simulink model "mrefrobotarm_previous_y_previous_u_previous_ref_cex_3b"  (R2018b)
settings: Solver=FixedStepAuto  StartTime=0.0  StopTime=20  RelTol=1e-3  AbsTol=1e-6
undefined symbols (not defined in the file or in its folder): cc, options
libraries: neural x462, simulink x2
(part 14 of 18)

== system mrefrobotarm_previous_y_previous_u_previous_ref_cex_3b/cex_m5/Layer 3/Delays 1 ==
  "p{3}" : Inport  PortDimensions=30
      mask Display: e = 0.06;c1 = [120 230 180]/255;c2 = ([120 230 180]+0)/(256+128);c3 = ([120 230 180]+128)/(256+128);patch([0 1 1 0],[0 0 1 1],c1);patch([0 1 1 1-e 1-e 0+e],[0 0 1 1-e 0+e 0+e],c2);patch([0 0 1 1-e 0+e 0+e],[0 1 1 1-e 1-e 0+e],c3);plot([0 1 1 0 0],[0 0 1 1 0]);
  mux : Mux  Inputs=1
      mask Display: e = 0.06;c1 = [120 150 230]/255;c2 = ([120 150 230]+0)/383;c3 = ([120 150 230]+128)/383;patch([0 1 1 0],[0 0 1 1],c1);patch([0 1 1 1-e 1-e 0+e],[0 0 1 1-e 0+e 0+e],c2);patch([0 0 1 1-e 0+e 0+e],[0 1 1 1-e 1-e 0+e],c3);plot([0 1 1 0 0],[0 0 1 1 0]);disp('Mux')
  "pd{3,2}" : Outport
      mask Display: e = 0.06;c1 = [120 230 180]/255;c2 = ([120 230 180]+0)/(256+128);c3 = ([120 230 180]+128)/(256+128);patch([0 1 1 0],[0 0 1 1],c1);patch([0 1 1 1-e 1-e 0+e],[0 0 1 1-e 0+e 0+e],c2);patch([0 0 1 1-e 0+e 0+e],[0 1 1 1-e 1-e 0+e],c3);plot([0 1 1 0 0],[0 0 1 1 0]);
  wires:
  "p{3}"/1 -> mux/1
  mux/1 -> "pd{3,2}"/1

== system mrefrobotarm_previous_y_previous_u_previous_ref_cex_3b/cex_m5/Layer 3/LW{3,2} ==
  "ad{3,2}" : Inport  PortDimensions=30
      mask Display: e = 0.06;c1 = [120 230 180]/255;c2 = ([120 230 180]+0)/(256+128);c3 = ([120 230 180]+128)/(256+128);patch([0 1 1 0],[0 0 1 1],c1);patch([0 1 1 1-e 1-e 0+e],[0 0 1 1-e 0+e 0+e],c2);patch([0 0 1 1-e 0+e 0+e],[0 1 1 1-e 1-e 0+e],c3);plot([0 1 1 0 0],[0 0 1 1 0]);
  "IW{3,2}(1,:)'" : Constant  Value=[0.50803666019963544808746291892020963132381439208984375;-0.729030644030080221540401907986961305141448974609375;0.09247581248743631798792108611451112665235996246337890625;-0.034331210467475899161815533489061635918915271759033203125;0.486684870445886763601350821772939525544643402099609375;0.7990123045007149205076757425558753311634063720703125;0.1682973469083234030474471865090890787541866302490234375;-0.474890180914950443824551484794938005506992340087890625;0.270457873152577799036322403480880893766880035400390625;-0.130728690312984008325969398356392048299312591552734375;-0.63017565134821751371418940834701061248779296875;0.28365242499360399097696472381358034908771514892578125;-0.11891322983694736781234979616783675737679004669189453125;0.444577906739277384229325207343208603560924530029296875;0.1091866209193628478590909480772097595036029815673828125;0.126623611089255960759913932633935473859310150146484375;0.88512666352133007041658174784970469772815704345703125;0.478777881050120923678292683689505793154239654541015625;0.4064587284632479313728481429279781877994537353515625;-0.317131905106795730642232911122846417129039764404296875;-0.7472199432531414498015465142088942229747772216796875;-0.7716850440813833866826598750776611268520355224609375;0.07278752047878193909280497564395773224532604217529296875;-0.12570824626491206021938751291600055992603302001953125;-0.2066677692862751436475576838347478769719600677490234375;0.8641321421683898496013398471404798328876495361328125;0.29316217307002201408749897382222115993499755859375;0.348121183619366003636486084360512904822826385498046875;0.10311848126639755474087678521755151450634002685546875;0.77075459933333989592796342549263499677181243896484375]
      mask Display: e = 0.06;c1 = [120 150 230]/255;c2 = ([120 150 230]+0)/383;c3 = ([120 150 230]+128)/383;patch([0 1 1 0],[0 0 1 1],c1);patch([0 1 1 1-e 1-e 0+e],[0 0 1 1-e 0+e 0+e],c2);patch([0 0 1 1-e 0+e 0+e],[0 1 1 1-e 1-e 0+e],c3);plot([0 1 1 0 0],[0 0 1 1 0]);disp('weights');
  Mux : Mux  Inputs=1
      mask Display: e = 0.06;c1 = [120 150 230]/255;c2 = ([120 150 230]+0)/383;c3 = ([120 150 230]+128)/383;patch([0 1 1 0],[0 0 1 1],c1);patch([0 1 1 1-e 1-e 0+e],[0 0 1 1-e 0+e 0+e],c2);patch([0 0 1 1-e 0+e 0+e],[0 1 1 1-e 1-e 0+e],c3);plot([0 1 1 0 0],[0 0 1 1 0]);disp('Mux');
  dotprod1 : neural/Weight Functions/dotprod
  "lz{3,2}" : Outport
      mask Display: e = 0.06;c1 = [120 230 180]/255;c2 = ([120 230 180]+0)/(256+128);c3 = ([120 230 180]+128)/(256+128);patch([0 1 1 0],[0 0 1 1],c1);patch([0 1 1 1-e 1-e 0+e],[0 0 1 1-e 0+e 0+e],c2);patch([0 0 1 1-e 0+e 0+e],[0 1 1 1-e 1-e 0+e],c3);plot([0 1 1 0 0],[0 0 1 1 0]);
  wires:
  "IW{3,2}(1,:)'"/1 -> dotprod1/1
  "ad{3,2}"/1 -> dotprod1/2
  dotprod1/1 -> Mux/1
  Mux/1 -> "lz{3,2}"/1

== system mrefrobotarm_previous_y_previous_u_previous_ref_cex_3b/no_cex/Layer 1/Delays 1 ==
  "p{1}" : Inport  PortDimensions=10
      mask Display: e = 0.06;c1 = [120 230 180]/255;c2 = ([120 230 180]+0)/(256+128);c3 = ([120 230 180]+128)/(256+128);patch([0 1 1 0],[0 0 1 1],c1);patch([0 1 1 1-e 1-e 0+e],[0 0 1 1-e 0+e 0+e],c2);patch([0 0 1 1-e 0+e 0+e],[0 1 1 1-e 1-e 0+e],c3);plot([0 1 1 0 0],[0 0 1 1 0]);
  mux : Mux  Inputs=1
      mask Display: e = 0.06;c1 = [120 150 230]/255;c2 = ([120 150 230]+0)/383;c3 = ([120 150 230]+128)/383;patch([0 1 1 0],[0 0 1 1],c1);patch([0 1 1 1-e 1-e 0+e],[0 0 1 1-e 0+e 0+e],c2);patch([0 0 1 1-e 0+e 0+e],[0 1 1 1-e 1-e 0+e],c3);plot([0 1 1 0 0],[0 0 1 1 0]);disp('Mux')
  "pd{1,1}" : Outport
      mask Display: e = 0.06;c1 = [120 230 180]/255;c2 = ([120 230 180]+0)/(256+128);c3 = ([120 230 180]+128)/(256+128);patch([0 1 1 0],[0 0 1 1],c1);patch([0 1 1 1-e 1-e 0+e],[0 0 1 1-e 0+e 0+e],c2);patch([0 0 1 1-e 0+e 0+e],[0 1 1 1-e 1-e 0+e],c3);plot([0 1 1 0 0],[0 0 1 1 0]);
  wires:
  "p{1}"/1 -> mux/1
  mux/1 -> "pd{1,1}"/1

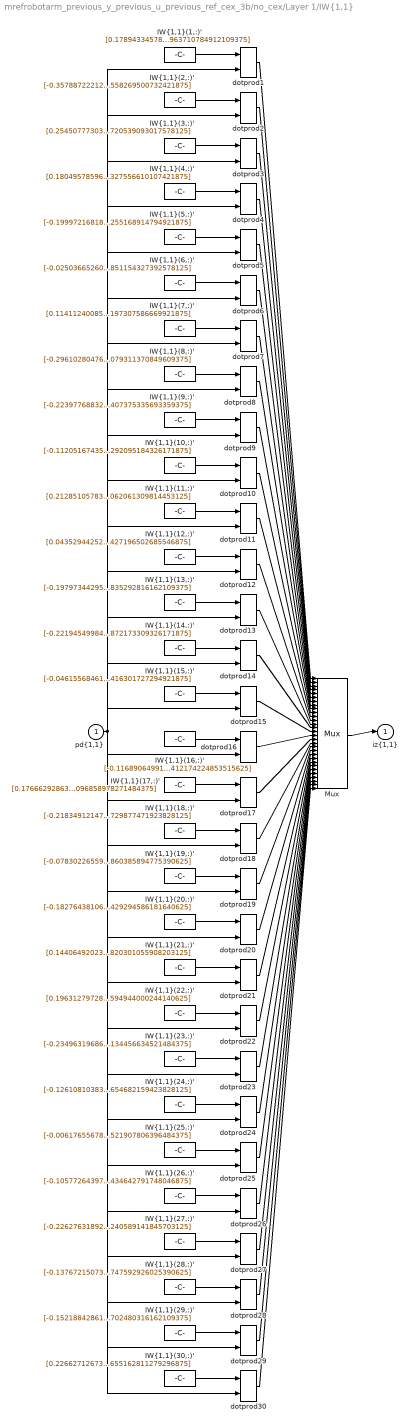
== system mrefrobotarm_previous_y_previous_u_previous_ref_cex_3b/no_cex/Layer 1/IW{1,1} ==
  "pd{1,1}" : Inport  PortDimensions=10
      mask Display: e = 0.06;c1 = [120 230 180]/255;c2 = ([120 230 180]+0)/(256+128);c3 = ([120 230 180]+128)/(256+128);patch([0 1 1 0],[0 0 1 1],c1);patch([0 1 1 1-e 1-e 0+e],[0 0 1 1-e 0+e 0+e],c2);patch([0 0 1 1-e 0+e 0+e],[0 1 1 1-e 1-e 0+e],c3);plot([0 1 1 0 0],[0 0 1 1 0]);
  "IW{1,1}(1,:)'" : Constant  Value=[0.1789433457845766017868527342216111719608306884765625;0.026806665156776932068538599196472205221652984619140625;-0.019425018864830494169648744673395412974059581756591796875;-0.08160374694861978472903984993536141701042652130126953125;-0.09141214122166922695367219375839340500533580780029296875;-0.0300317987322644870673560291152170975692570209503173828125;-0.28242027541455028138983607277623377740383148193359375;0.131111008237114468055750649000401608645915985107421875;-0.1895896042370200651472345043657696805894374847412109375;0.2425039454857501330931057736961520276963710784912109375]
      mask Display: e = 0.06;c1 = [120 150 230]/255;c2 = ([120 150 230]+0)/383;c3 = ([120 150 230]+128)/383;patch([0 1 1 0],[0 0 1 1],c1);patch([0 1 1 1-e 1-e 0+e],[0 0 1 1-e 0+e 0+e],c2);patch([0 0 1 1-e 0+e 0+e],[0 1 1 1-e 1-e 0+e],c3);plot([0 1 1 0 0],[0 0 1 1 0]);disp('Weights');
  "IW{1,1}(10,:)'" : Constant  Value=[-0.11205167435669681486043458562562591396272182464599609375;0.3571497785474593289478661972680129110813140869140625;-0.2471594181194160799730497046766686253249645233154296875;0.0269727210263034818116256730036184308119118213653564453125;0.333375233420288186181323908385820686817169189453125;-0.3923415376813588206772465127869509160518646240234375;0.10451408189524002967374372019548900425434112548828125;-0.06697052425982270851267941225160029716789722442626953125;-0.08640964459355114646310624948455370031297206878662109375;-0.39109382895870126173321068563382141292095184326171875]
      mask Display: e = 0.06;c1 = [120 150 230]/255;c2 = ([120 150 230]+0)/383;c3 = ([120 150 230]+128)/383;patch([0 1 1 0],[0 0 1 1],c1);patch([0 1 1 1-e 1-e 0+e],[0 0 1 1-e 0+e 0+e],c2);patch([0 0 1 1-e 0+e 0+e],[0 1 1 1-e 1-e 0+e],c3);plot([0 1 1 0 0],[0 0 1 1 0]);disp('Weights');
  "IW{1,1}(11,:)'" : Constant  Value=[0.2128510578334973646352779041990288533270359039306640625;-0.202231663792214522157308920213836245238780975341796875;0.0248759940897357034739201253614737652242183685302734375;-0.15238132615766508681787172463373281061649322509765625;0.01341935499692491380596681693759819609113037586212158203125;0.333773414996746620175827047205530107021331787109375;-0.12205302921810114169520744553665281273424625396728515625;0.154445274700418855307049170733080245554447174072265625;-0.0299658607885634718781542318311039707623422145843505859375;0.1513989913513389684585064287603017874062061309814453125]
      mask Display: e = 0.06;c1 = [120 150 230]/255;c2 = ([120 150 230]+0)/383;c3 = ([120 150 230]+128)/383;patch([0 1 1 0],[0 0 1 1],c1);patch([0 1 1 1-e 1-e 0+e],[0 0 1 1-e 0+e 0+e],c2);patch([0 0 1 1-e 0+e 0+e],[0 1 1 1-e 1-e 0+e],c3);plot([0 1 1 0 0],[0 0 1 1 0]);disp('Weights');
  "IW{1,1}(12,:)'" : Constant  Value=[0.04352944252029027072392608488371479324996471405029296875;-0.4145342324684342383278590205009095370769500732421875;0.215269820769206976507348372251726686954498291015625;0.16656367985601061576517167850397527217864990234375;-0.023581251549110941734266333469349774532020092010498046875;0.08572964794493535822805796442480641417205333709716796875;-0.1958135172033455273510327288022381253540515899658203125;-0.1625056502497410904073404935843427665531635284423828125;0.251217425233158042630066120182164013385772705078125;-0.1069272106474794536978834003093652427196502685546875]
      mask Display: e = 0.06;c1 = [120 150 230]/255;c2 = ([120 150 230]+0)/383;c3 = ([120 150 230]+128)/383;patch([0 1 1 0],[0 0 1 1],c1);patch([0 1 1 1-e 1-e 0+e],[0 0 1 1-e 0+e 0+e],c2);patch([0 0 1 1-e 0+e 0+e],[0 1 1 1-e 1-e 0+e],c3);plot([0 1 1 0 0],[0 0 1 1 0]);disp('Weights');
  "IW{1,1}(13,:)'" : Constant  Value=[-0.1979734429534960316043878947311895899474620819091796875;0.184541564617396514069724844375741668045520782470703125;-0.0638366095873931505000342667699442245066165924072265625;0.2121216584407361882558262777820345945656299591064453125;-0.1380891994715965076512276255016331560909748077392578125;0.038970800909377711906955710219335742294788360595703125;0.1056185799492942722910271413638838566839694976806640625;-0.150221719826857891266769229332567192614078521728515625;-0.2463272007812304931206881519756279885768890380859375;0.217176977670956394828039037747657857835292816162109375]
      mask Display: e = 0.06;c1 = [120 150 230]/255;c2 = ([120 150 230]+0)/383;c3 = ([120 150 230]+128)/383;patch([0 1 1 0],[0 0 1 1],c1);patch([0 1 1 1-e 1-e 0+e],[0 0 1 1-e 0+e 0+e],c2);patch([0 0 1 1-e 0+e 0+e],[0 1 1 1-e 1-e 0+e],c3);plot([0 1 1 0 0],[0 0 1 1 0]);disp('Weights');
  "IW{1,1}(14,:)'" : Constant  Value=[-0.2219454998402757561759557347613736055791378021240234375;-0.03146157022389335644607655240179155953228473663330078125;0.251007319128800698848635875037871301174163818359375;-0.0716759659946031302268920626374892890453338623046875;-0.0172769424599281511134574174093359033577144145965576171875;0.187315939375391149468441653880290687084197998046875;0.1900738665719299003153963667500647716224193572998046875;0.256287588268780563982573994508129544556140899658203125;-0.12311552872518909118593199991664732806384563446044921875;0.083687737575868836881198831179062835872173309326171875]
      mask Display: e = 0.06;c1 = [120 150 230]/255;c2 = ([120 150 230]+0)/383;c3 = ([120 150 230]+128)/383;patch([0 1 1 0],[0 0 1 1],c1);patch([0 1 1 1-e 1-e 0+e],[0 0 1 1-e 0+e 0+e],c2);patch([0 0 1 1-e 0+e 0+e],[0 1 1 1-e 1-e 0+e],c3);plot([0 1 1 0 0],[0 0 1 1 0]);disp('Weights');
  "IW{1,1}(15,:)'" : Constant  Value=[-0.046155684619317384476122612113613286055624485015869140625;-0.1501347766892376645042617155922926031053066253662109375;0.00923054671975952721607594497754689655266702175140380859375;-0.263036162746853541261060627221013419330120086669921875;-0.232797656826339238733680758741684257984161376953125;-0.20261136681460356623318830315838567912578582763671875;0.051737147633385383027615489481831900775432586669921875;-0.2097569798040830324481476054643280804157257080078125;0.1810701944794087248080671770367189310491085052490234375;-0.037977663494814066502680560688531841151416301727294921875]
      mask Display: e = 0.06;c1 = [120 150 230]/255;c2 = ([120 150 230]+0)/383;c3 = ([120 150 230]+128)/383;patch([0 1 1 0],[0 0 1 1],c1);patch([0 1 1 1-e 1-e 0+e],[0 0 1 1-e 0+e 0+e],c2);patch([0 0 1 1-e 0+e 0+e],[0 1 1 1-e 1-e 0+e],c3);plot([0 1 1 0 0],[0 0 1 1 0]);disp('Weights');
  "IW{1,1}(16,:)'" : Constant  Value=[-0.11689064991597501730336006176003138534724712371826171875;0.1948274101793631418733099280871101655066013336181640625;0.245143937349593776797718192028696648776531219482421875;0.06314433664036896154403422087852959521114826202392578125;-0.1710716489566988240955680566912633366882801055908203125;0.228635751900371164690994874035823158919811248779296875;0.167954804626501530417925778237986378371715545654296875;-0.1360225837338669696574555700863129459321498870849609375;0.1710850798697334529396840707704541273415088653564453125;-0.03517706195236515454016767989742220379412174224853515625]
      mask Display: e = 0.06;c1 = [120 150 230]/255;c2 = ([120 150 230]+0)/383;c3 = ([120 150 230]+128)/383;patch([0 1 1 0],[0 0 1 1],c1);patch([0 1 1 1-e 1-e 0+e],[0 0 1 1-e 0+e 0+e],c2);patch([0 0 1 1-e 0+e 0+e],[0 1 1 1-e 1-e 0+e],c3);plot([0 1 1 0 0],[0 0 1 1 0]);disp('Weights');
  "IW{1,1}(17,:)'" : Constant  Value=[0.1766629286340325732940215175403864122927188873291015625;-0.07924000184714556638265747778859804384410381317138671875;-0.079307885697641300470905889596906490623950958251953125;-0.1959224066965960242558963955161743797361850738525390625;0.1156529952522807602743881716378382407128810882568359375;0.00787969713280355955886680163757773698307573795318603515625;0.042693454259183853671810737751002307049930095672607421875;-0.2093969688941783591218381843646056950092315673828125;-0.1737244673605020661710796048282645642757415771484375;-0.30776382007785529903998167355894111096858978271484375]
      mask Display: e = 0.06;c1 = [120 150 230]/255;c2 = ([120 150 230]+0)/383;c3 = ([120 150 230]+128)/383;patch([0 1 1 0],[0 0 1 1],c1);patch([0 1 1 1-e 1-e 0+e],[0 0 1 1-e 0+e 0+e],c2);patch([0 0 1 1-e 0+e 0+e],[0 1 1 1-e 1-e 0+e],c3);plot([0 1 1 0 0],[0 0 1 1 0]);disp('Weights');
  "IW{1,1}(18,:)'" : Constant  Value=[-0.2183491214766035692917967026005499064922332763671875;0.064228498311528825492899841265170834958553314208984375;-0.061951741605276833269044800545088946819305419921875;0.0980483298401862712889709428054629825055599212646484375;-0.1940715279329147946452138739914516918361186981201171875;0.100554472875109379703673084804904647171497344970703125;0.05512572940682851363458638616066309623420238494873046875;-0.2225697983573027005643751863317447714507579803466796875;0.307695093952117415536662292652181349694728851318359375;0.035102615659615206411547916331983287818729877471923828125]
      mask Display: e = 0.06;c1 = [120 150 230]/255;c2 = ([120 150 230]+0)/383;c3 = ([120 150 230]+128)/383;patch([0 1 1 0],[0 0 1 1],c1);patch([0 1 1 1-e 1-e 0+e],[0 0 1 1-e 0+e 0+e],c2);patch([0 0 1 1-e 0+e 0+e],[0 1 1 1-e 1-e 0+e],c3);plot([0 1 1 0 0],[0 0 1 1 0]);disp('Weights');
  "IW{1,1}(19,:)'" : Constant  Value=[-0.078302265597536335750561420354642905294895172119140625;-0.11015731653471379225539550361645524390041828155517578125;0.070372247422889111501120851244195364415645599365234375;-0.07371385722816987950967160259096999652683734893798828125;0.2498389657291748833234379389978130348026752471923828125;-0.14478671437019630108267165269353426992893218994140625;0.3213022509194900511175774227012880146503448486328125;0.014213136324984949887539897872557048685848712921142578125;-0.209759210724774380896207048863288946449756622314453125;-0.13789802555820040996792386067681945860385894775390625]
      mask Display: e = 0.06;c1 = [120 150 230]/255;c2 = ([120 150 230]+0)/383;c3 = ([120 150 230]+128)/383;patch([0 1 1 0],[0 0 1 1],c1);patch([0 1 1 1-e 1-e 0+e],[0 0 1 1-e 0+e 0+e],c2);patch([0 0 1 1-e 0+e 0+e],[0 1 1 1-e 1-e 0+e],c3);plot([0 1 1 0 0],[0 0 1 1 0]);disp('Weights');
  "IW{1,1}(2,:)'" : Constant  Value=[-0.357887222121373971273072811527526937425136566162109375;-0.1701508970623704930513753197374171577394008636474609375;0.1283995799451636832255729814278311096131801605224609375;0.027882319431207010229645248955421266146004199981689453125;0.2413367899208160860524685631389729678630828857421875;-0.08829939749269695437039473517870646901428699493408203125;-0.059645223459835527979322478131507523357868194580078125;-0.1817708312802679693209739753001485951244831085205078125;-0.202751405688736785482007007885840721428394317626953125;0.036121615813504197312067134362223441712558269500732421875]
      mask Display: e = 0.06;c1 = [120 150 230]/255;c2 = ([120 150 230]+0)/383;c3 = ([120 150 230]+128)/383;patch([0 1 1 0],[0 0 1 1],c1);patch([0 1 1 1-e 1-e 0+e],[0 0 1 1-e 0+e 0+e],c2);patch([0 0 1 1-e 0+e 0+e],[0 1 1 1-e 1-e 0+e],c3);plot([0 1 1 0 0],[0 0 1 1 0]);disp('Weights');
  "IW{1,1}(20,:)'" : Constant  Value=[-0.1827643810609429209090848189589451067149639129638671875;0.429780420918997874135669690076611004769802093505859375;0.04752296112356881041538514409694471396505832672119140625;-0.051704435533531163671217001365221221931278705596923828125;0.09194866005832495747807087127512204460799694061279296875;-0.378826441233361788096800637504202313721179962158203125;-0.032643642152327199956740599873228347860276699066162109375;-0.035924345859773477995791068906328291632235050201416015625;-0.0821961773385673499792147822518018074333667755126953125;-0.1229117568782160108131762399352737702429294586181640625]
      mask Display: e = 0.06;c1 = [120 150 230]/255;c2 = ([120 150 230]+0)/383;c3 = ([120 150 230]+128)/383;patch([0 1 1 0],[0 0 1 1],c1);patch([0 1 1 1-e 1-e 0+e],[0 0 1 1-e 0+e 0+e],c2);patch([0 0 1 1-e 0+e 0+e],[0 1 1 1-e 1-e 0+e],c3);plot([0 1 1 0 0],[0 0 1 1 0]);disp('Weights');
  "IW{1,1}(21,:)'" : Constant  Value=[0.144064920235662696779144198444555513560771942138671875;0.056739780550756180321769761576433666050434112548828125;0.1869901994016132940057417499701841734349727630615234375;-0.1647949003581190841050130302392062731087207794189453125;-0.237382679487966596898473881083191372454166412353515625;0.25368592107000653701476267087855376303195953369140625;-0.234657572045289197770756572936079464852809906005859375;0.021587502157350169085248126066289842128753662109375;0.23838937978631380421035146355279721319675445556640625;-0.002599061752152885713951224744278079015202820301055908203125]
      mask Display: e = 0.06;c1 = [120 150 230]/255;c2 = ([120 150 230]+0)/383;c3 = ([120 150 230]+128)/383;patch([0 1 1 0],[0 0 1 1],c1);patch([0 1 1 1-e 1-e 0+e],[0 0 1 1-e 0+e 0+e],c2);patch([0 0 1 1-e 0+e 0+e],[0 1 1 1-e 1-e 0+e],c3);plot([0 1 1 0 0],[0 0 1 1 0]);disp('Weights');
  "IW{1,1}(22,:)'" : Constant  Value=[0.196312797288851148547195180071867071092128753662109375;-0.052003440136825181128177320033501018770039081573486328125;-0.271537484269043394302656224681413732469081878662109375;-0.08952689103963186456613954078420647419989109039306640625;-0.03695367511956813844076208397382288239896297454833984375;0.00447587075779976202583032574011667747981846332550048828125;0.2592011849893742780892580412910319864749908447265625;-0.088946395220038609874535495691816322505474090576171875;0.0322691823643851682934524660595343448221683502197265625;0.30695137976644348842825138490297831594944000244140625]
      mask Display: e = 0.06;c1 = [120 150 230]/255;c2 = ([120 150 230]+0)/383;c3 = ([120 150 230]+128)/383;patch([0 1 1 0],[0 0 1 1],c1);patch([0 1 1 1-e 1-e 0+e],[0 0 1 1-e 0+e 0+e],c2);patch([0 0 1 1-e 0+e 0+e],[0 1 1 1-e 1-e 0+e],c3);plot([0 1 1 0 0],[0 0 1 1 0]);disp('Weights');
  "IW{1,1}(23,:)'" : Constant  Value=[-0.2349631968647795388083210355034680105745792388916015625;-0.1764143763037677448135553959218668751418590545654296875;0.2349121078796777284392049978123395703732967376708984375;0.09797592905204242919037227466105832718312740325927734375;0.27541249925572675039120440487749874591827392578125;-0.00667307854933686661613734258935437537729740142822265625;-0.0863088887077549105075746638249256648123264312744140625;-0.049254487681551224753651041510238428600132465362548828125;0.3119811716961577996443111260305158793926239013671875;-0.1301709247348719900028157780980109237134456634521484375]
      mask Display: e = 0.06;c1 = [120 150 230]/255;c2 = ([120 150 230]+0)/383;c3 = ([120 150 230]+128)/383;patch([0 1 1 0],[0 0 1 1],c1);patch([0 1 1 1-e 1-e 0+e],[0 0 1 1-e 0+e 0+e],c2);patch([0 0 1 1-e 0+e 0+e],[0 1 1 1-e 1-e 0+e],c3);plot([0 1 1 0 0],[0 0 1 1 0]);disp('Weights');
  "IW{1,1}(24,:)'" : Constant  Value=[-0.126108103838845353461550757856457494199275970458984375;0.08453501177616129513836540354532189667224884033203125;-0.1709620737039248272726155164491501636803150177001953125;0.291184483266852811578218052090960554778575897216796875;0.11522387540724605969888472145612468011677265167236328125;0.27025016099325138707598625842365436255931854248046875;0.115017676269625723772804803957114927470684051513671875;0.06893159212255894896514973879675380885601043701171875;0.09231217475138053796257509020506404340267181396484375;0.1257462335265127351124903043455560691654682159423828125]
      mask Display: e = 0.06;c1 = [120 150 230]/255;c2 = ([120 150 230]+0)/383;c3 = ([120 150 230]+128)/383;patch([0 1 1 0],[0 0 1 1],c1);patch([0 1 1 1-e 1-e 0+e],[0 0 1 1-e 0+e 0+e],c2);patch([0 0 1 1-e 0+e 0+e],[0 1 1 1-e 1-e 0+e],c3);plot([0 1 1 0 0],[0 0 1 1 0]);disp('Weights');
  "IW{1,1}(25,:)'" : Constant  Value=[-0.00617655678054580652147631525394899654202163219451904296875;0.158550050715132895273740132324746809899806976318359375;0.18860048113506466815891826627193950116634368896484375;-0.016879223596091640080540940971332020126283168792724609375;-0.1887910208933633315897537841010489501059055328369140625;0.1272457432851887559888126588703016750514507293701171875;-0.018568139538292789680884453673570533283054828643798828125;0.2719728918008812446061028822441585361957550048828125;0.1140621157238612404238864428407396189868450164794921875;-0.2380940842603967710910950472680269740521907806396484375]
      mask Display: e = 0.06;c1 = [120 150 230]/255;c2 = ([120 150 230]+0)/383;c3 = ([120 150 230]+128)/383;patch([0 1 1 0],[0 0 1 1],c1);patch([0 1 1 1-e 1-e 0+e],[0 0 1 1-e 0+e 0+e],c2);patch([0 0 1 1-e 0+e 0+e],[0 1 1 1-e 1-e 0+e],c3);plot([0 1 1 0 0],[0 0 1 1 0]);disp('Weights');
  "IW{1,1}(26,:)'" : Constant  Value=[-0.105772643970521940115503412016551010310649871826171875;0.1782055718246454978359594178982661105692386627197265625;-0.257768734053310577536421988043002784252166748046875;-0.12118741242321341700094450288816005922853946685791015625;0.10799318799709652083596012062116642482578754425048828125;0.032415029855224826438320206989374128170311450958251953125;0.23392792477851431787172487020143307745456695556640625;0.048627216784484859901649400626411079429090023040771484375;-0.07777159955391781120948024863537284545600414276123046875;-0.066068946728559563297267231973819434642791748046875]
      mask Display: e = 0.06;c1 = [120 150 230]/255;c2 = ([120 150 230]+0)/383;c3 = ([120 150 230]+128)/383;patch([0 1 1 0],[0 0 1 1],c1);patch([0 1 1 1-e 1-e 0+e],[0 0 1 1-e 0+e 0+e],c2);patch([0 0 1 1-e 0+e 0+e],[0 1 1 1-e 1-e 0+e],c3);plot([0 1 1 0 0],[0 0 1 1 0]);disp('Weights');
  "IW{1,1}(27,:)'" : Constant  Value=[-0.2262763189227159077443474188839900307357311248779296875;0.2283819320597203772482686190414824523031711578369140625;-0.046330569948930359902572462260650354437530040740966796875;-0.21556632228014915853009370039217174053192138671875;-0.024471900852634960454867751877827686257660388946533203125;-0.061310669133914065531687498378232703544199466705322265625;0.1926380354105947934062470494609442539513111114501953125;0.2138008717117891588355149679046007804572582244873046875;0.2402187286512235953050975467704120092093944549560546875;0.004683890847436260503056093540408255648799240589141845703125]
      mask Display: e = 0.06;c1 = [120 150 230]/255;c2 = ([120 150 230]+0)/383;c3 = ([120 150 230]+128)/383;patch([0 1 1 0],[0 0 1 1],c1);patch([0 1 1 1-e 1-e 0+e],[0 0 1 1-e 0+e 0+e],c2);patch([0 0 1 1-e 0+e 0+e],[0 1 1 1-e 1-e 0+e],c3);plot([0 1 1 0 0],[0 0 1 1 0]);disp('Weights');
  "IW{1,1}(28,:)'" : Constant  Value=[-0.1376721507398574739777785680416855029761791229248046875;0.1357305892334177144231688316722284071147441864013671875;0.10902662094067107345640721405288786627352237701416015625;-0.0209302692967432597825894191601037164218723773956298828125;0.1596193252357711311884003180239233188331127166748046875;-0.22463253929018323074018326224177144467830657958984375;-0.126742784051142420853608427933068014681339263916015625;0.1520246488067715506797838997954386286437511444091796875;0.2181396982129823192142481502742157317698001861572265625;-0.0472266865883811670645542335478239692747592926025390625]
      mask Display: e = 0.06;c1 = [120 150 230]/255;c2 = ([120 150 230]+0)/383;c3 = ([120 150 230]+128)/383;patch([0 1 1 0],[0 0 1 1],c1);patch([0 1 1 1-e 1-e 0+e],[0 0 1 1-e 0+e 0+e],c2);patch([0 0 1 1-e 0+e 0+e],[0 1 1 1-e 1-e 0+e],c3);plot([0 1 1 0 0],[0 0 1 1 0]);disp('Weights');
  "IW{1,1}(29,:)'" : Constant  Value=[-0.1521884286183979029249968561998684890568256378173828125;-0.045825061815970465073366568731216830201447010040283203125;0.075552021378081202218623957378440536558628082275390625;-0.185262385097363424524274932991829700767993927001953125;0.151250917067363932488888167426921427249908447265625;-0.1412092387151698547054223809027462266385555267333984375;-0.08681829974009762362907594024363788776099681854248046875;-0.2248735479200896503204631926564616151154041290283203125;-0.1651995887555126885093415012306650169193744659423828125;0.157553780756952865882425385279930196702480316162109375]
      mask Display: e = 0.06;c1 = [120 150 230]/255;c2 = ([120 150 230]+0)/383;c3 = ([120 150 230]+128)/383;patch([0 1 1 0],[0 0 1 1],c1);patch([0 1 1 1-e 1-e 0+e],[0 0 1 1-e 0+e 0+e],c2);patch([0 0 1 1-e 0+e 0+e],[0 1 1 1-e 1-e 0+e],c3);plot([0 1 1 0 0],[0 0 1 1 0]);disp('Weights');
  "IW{1,1}(3,:)'" : Constant  Value=[0.2545077730308322738750348435132764279842376708984375;0.040200772337387093158245221502511412836611270904541015625;0.1688552759835511007935338056995533406734466552734375;0.2275439474123589767007302953061298467218875885009765625;0.238416378071425294482565959697240032255649566650390625;0.1413290648624935530452972898274310864508152008056640625;0.1057585717371296307742767339732381515204906463623046875;0.1334076779718362526505615051064523868262767791748046875;0.120305182199565041667455034257727675139904022216796875;0.11598616375682953283376974695784156210720539093017578125]
      mask Display: e = 0.06;c1 = [120 150 230]/255;c2 = ([120 150 230]+0)/383;c3 = ([120 150 230]+128)/383;patch([0 1 1 0],[0 0 1 1],c1);patch([0 1 1 1-e 1-e 0+e],[0 0 1 1-e 0+e 0+e],c2);patch([0 0 1 1-e 0+e 0+e],[0 1 1 1-e 1-e 0+e],c3);plot([0 1 1 0 0],[0 0 1 1 0]);disp('Weights');
  "IW{1,1}(30,:)'" : Constant  Value=[0.2266271267387724719366559611444245092570781707763671875;0.1400905747425138792028320722238277085125446319580078125;-0.1118692708200293151055149110106867738068103790283203125;0.20125294810015048607709786665509454905986785888671875;-0.0186267634903538349677720731278895982541143894195556640625;-0.200639624098857660694505966603173874318599700927734375;-0.09615771229638904460390591566465445794165134429931640625;-0.177214543927699696990174516031402163207530975341796875;0.03191830542659655767234738732440746389329433441162109375;0.2669655305019122959464539235341362655162811279296875]
      mask Display: e = 0.06;c1 = [120 150 230]/255;c2 = ([120 150 230]+0)/383;c3 = ([120 150 230]+128)/383;patch([0 1 1 0],[0 0 1 1],c1);patch([0 1 1 1-e 1-e 0+e],[0 0 1 1-e 0+e 0+e],c2);patch([0 0 1 1-e 0+e 0+e],[0 1 1 1-e 1-e 0+e],c3);plot([0 1 1 0 0],[0 0 1 1 0]);disp('Weights');
  "IW{1,1}(4,:)'" : Constant  Value=[0.1804957859696745270383644310641102492809295654296875;-0.2288584972184532217998054193230927921831607818603515625;0.1818629338165111963832032415666617453098297119140625;-0.037952073411335406072364406782071455381810665130615234375;-0.00539871852212082947719551384579972364008426666259765625;0.182786368740827043222196834904025308787822723388671875;-0.055300908131749697271839494305822881869971752166748046875;-0.1474442788239329893418272376948152668774127960205078125;-0.27933026497486468375797130647697485983371734619140625;0.132250800721111338997815209950204007327556610107421875]
      mask Display: e = 0.06;c1 = [120 150 230]/255;c2 = ([120 150 230]+0)/383;c3 = ([120 150 230]+128)/383;patch([0 1 1 0],[0 0 1 1],c1);patch([0 1 1 1-e 1-e 0+e],[0 0 1 1-e 0+e 0+e],c2);patch([0 0 1 1-e 0+e 0+e],[0 1 1 1-e 1-e 0+e],c3);plot([0 1 1 0 0],[0 0 1 1 0]);disp('Weights');
  "IW{1,1}(5,:)'" : Constant  Value=[-0.19997216818005469907149063146789558231830596923828125;-0.1629615728772902116805454397763242013752460479736328125;-0.1088061302365657123658593263826332986354827880859375;0.051130930700108122299862856152685708366334438323974609375;-0.023722808228792462148515340913945692591369152069091796875;0.05171942315686968438814830051342141814529895782470703125;-0.172023141245443100810774694764404557645320892333984375;-0.2044816274455876214943828017567284405231475830078125;0.166303750238228686963992686287383548915386199951171875;-0.139186544766161268693593910938943736255168914794921875]
      mask Display: e = 0.06;c1 = [120 150 230]/255;c2 = ([120 150 230]+0)/383;c3 = ([120 150 230]+128)/383;patch([0 1 1 0],[0 0 1 1],c1);patch([0 1 1 1-e 1-e 0+e],[0 0 1 1-e 0+e 0+e],c2);patch([0 0 1 1-e 0+e 0+e],[0 1 1 1-e 1-e 0+e],c3);plot([0 1 1 0 0],[0 0 1 1 0]);disp('Weights');
  "IW{1,1}(6,:)'" : Constant  Value=[-0.025036652606763708239778765118899173103272914886474609375;-0.004459660997023274543737958452993552782572805881500244140625;0.06640274816857501261058160935135674662888050079345703125;-0.213061242876234679943792116318945772945880889892578125;0.1292954929203400105119925456165219657123088836669921875;-0.1347784484203936317125993582521914504468441009521484375;-0.2359879168296239171365158426851849071681499481201171875;-0.06529033806976369813668270580819807946681976318359375;-0.1443014597905320772763815284633892588317394256591796875;0.08876780395364276821101867653851513750851154327392578125]
      mask Display: e = 0.06;c1 = [120 150 230]/255;c2 = ([120 150 230]+0)/383;c3 = ([120 150 230]+128)/383;patch([0 1 1 0],[0 0 1 1],c1);patch([0 1 1 1-e 1-e 0+e],[0 0 1 1-e 0+e 0+e],c2);patch([0 0 1 1-e 0+e 0+e],[0 1 1 1-e 1-e 0+e],c3);plot([0 1 1 0 0],[0 0 1 1 0]);disp('Weights');
  "IW{1,1}(7,:)'" : Constant  Value=[0.114112400854734563626635690525290556252002716064453125;-0.0719764852942859356677018922709976322948932647705078125;0.21942076440832936068403569151996634900569915771484375;0.20872027523270497706420201211585663259029388427734375;0.042791134284794786479810824175729067064821720123291015625;0.01219358252673974352120467301574535667896270751953125;0.103149329692884206277625480652204714715480804443359375;0.2155964323288774020515035090284072794020175933837890625;-0.11201445164094690765121953290872625075280666351318359375;0.267689621647867692644240378285758197307586669921875]
      mask Display: e = 0.06;c1 = [120 150 230]/255;c2 = ([120 150 230]+0)/383;c3 = ([120 150 230]+128)/383;patch([0 1 1 0],[0 0 1 1],c1);patch([0 1 1 1-e 1-e 0+e],[0 0 1 1-e 0+e 0+e],c2);patch([0 0 1 1-e 0+e 0+e],[0 1 1 1-e 1-e 0+e],c3);plot([0 1 1 0 0],[0 0 1 1 0]);disp('Weights');
  "IW{1,1}(8,:)'" : Constant  Value=[-0.296102804766170513151024579201475717127323150634765625;-0.074634028193786450255942099829553626477718353271484375;-0.2385550334875161937464582706525106914341449737548828125;-0.205611704822805829717680126123013906180858612060546875;0.0525654127691315142811845362302847206592559814453125;-0.14543344256929569002778634967398829758167266845703125;0.1567883935266303208067029117955826222896575927734375;0.17216661658090737230253353118314407765865325927734375;-0.0903177999287110566672964750978280790150165557861328125;-0.05251414846928435797845935439909226261079311370849609375]
      mask Display: e = 0.06;c1 = [120 150 230]/255;c2 = ([120 150 230]+0)/383;c3 = ([120 150 230]+128)/383;patch([0 1 1 0],[0 0 1 1],c1);patch([0 1 1 1-e 1-e 0+e],[0 0 1 1-e 0+e 0+e],c2);patch([0 0 1 1-e 0+e 0+e],[0 1 1 1-e 1-e 0+e],c3);plot([0 1 1 0 0],[0 0 1 1 0]);disp('Weights');
  "IW{1,1}(9,:)'" : Constant  Value=[-0.223977688326731871892860681327874772250652313232421875;-0.1882936136938099525028889047462143935263156890869140625;-0.0257945746484941167142590501271115499548614025115966796875;0.07815143539481080037223392764644813723862171173095703125;0.03562614155169104013243241979580488987267017364501953125;-0.037321098578910867626934333429744583554565906524658203125;-0.280712738764397007340534173636115156114101409912109375;0.32608983885085562892669486245722509920597076416015625;0.05207556045307785985709614351435448043048381805419921875;-0.017162587892261237099145176898673526011407375335693359375]
      mask Display: e = 0.06;c1 = [120 150 230]/255;c2 = ([120 150 230]+0)/383;c3 = ([120 150 230]+128)/383;patch([0 1 1 0],[0 0 1 1],c1);patch([0 1 1 1-e 1-e 0+e],[0 0 1 1-e 0+e 0+e],c2);patch([0 0 1 1-e 0+e 0+e],[0 1 1 1-e 1-e 0+e],c3);plot([0 1 1 0 0],[0 0 1 1 0]);disp('Weights');
  Mux : Mux  Inputs=30
      mask Display: e = 0.06;c1 = [120 150 230]/255;c2 = ([120 150 230]+0)/383;c3 = ([120 150 230]+128)/383;patch([0 1 1 0],[0 0 1 1],c1);patch([0 1 1 1-e 1-e 0+e],[0 0 1 1-e 0+e 0+e],c2);patch([0 0 1 1-e 0+e 0+e],[0 1 1 1-e 1-e 0+e],c3);plot([0 1 1 0 0],[0 0 1 1 0]);disp('Mux');
  dotprod{1..30} (30 alike) : neural/Weight Functions/dotprod
  "iz{1,1}" : Outport
      mask Display: e = 0.06;c1 = [120 230 180]/255;c2 = ([120 230 180]+0)/(256+128);c3 = ([120 230 180]+128)/(256+128);patch([0 1 1 0],[0 0 1 1],c1);patch([0 1 1 1-e 1-e 0+e],[0 0 1 1-e 0+e 0+e],c2);patch([0 0 1 1-e 0+e 0+e],[0 1 1 1-e 1-e 0+e],c3);plot([0 1 1 0 0],[0 0 1 1 0]);
  wires:
  "IW{1,1}(1,:)'"/1 -> dotprod1/1
  "pd{1,1}"/1 -> dotprod1/2, dotprod2/2, dotprod3/2, dotprod4/2, dotprod5/2, dotprod6/2, dotprod7/2, dotprod8/2, dotprod9/2, dotprod10/2, dotprod11/2, dotprod12/2, dotprod13/2, dotprod14/2, dotprod15/2, dotprod16/2, dotprod17/2, dotprod18/2, dotprod19/2, dotprod20/2, dotprod21/2, dotprod22/2, dotprod23/2, dotprod24/2, dotprod25/2, dotprod26/2, dotprod27/2, dotprod28/2, dotprod29/2, dotprod30/2
  dotprod1/1 -> Mux/1
  "IW{1,1}(2,:)'"/1 -> dotprod2/1
  dotprod2/1 -> Mux/2
  "IW{1,1}(3,:)'"/1 -> dotprod3/1
  dotprod3/1 -> Mux/3
  "IW{1,1}(4,:)'"/1 -> dotprod4/1
  dotprod4/1 -> Mux/4
  "IW{1,1}(5,:)'"/1 -> dotprod5/1
  dotprod5/1 -> Mux/5
  "IW{1,1}(6,:)'"/1 -> dotprod6/1
  dotprod6/1 -> Mux/6
  "IW{1,1}(7,:)'"/1 -> dotprod7/1
  dotprod7/1 -> Mux/7
  "IW{1,1}(8,:)'"/1 -> dotprod8/1
  dotprod8/1 -> Mux/8
  "IW{1,1}(9,:)'"/1 -> dotprod9/1
  dotprod9/1 -> Mux/9
  "IW{1,1}(10,:)'"/1 -> dotprod10/1
  dotprod10/1 -> Mux/10
  "IW{1,1}(11,:)'"/1 -> dotprod11/1
  dotprod11/1 -> Mux/11
  "IW{1,1}(12,:)'"/1 -> dotprod12/1
  dotprod12/1 -> Mux/12
  "IW{1,1}(13,:)'"/1 -> dotprod13/1
  dotprod13/1 -> Mux/13
  "IW{1,1}(14,:)'"/1 -> dotprod14/1
  dotprod14/1 -> Mux/14
  "IW{1,1}(15,:)'"/1 -> dotprod15/1
  dotprod15/1 -> Mux/15
  "IW{1,1}(16,:)'"/1 -> dotprod16/1
  dotprod16/1 -> Mux/16
  "IW{1,1}(17,:)'"/1 -> dotprod17/1
  dotprod17/1 -> Mux/17
  "IW{1,1}(18,:)'"/1 -> dotprod18/1
  dotprod18/1 -> Mux/18
  "IW{1,1}(19,:)'"/1 -> dotprod19/1
  dotprod19/1 -> Mux/19
  "IW{1,1}(20,:)'"/1 -> dotprod20/1
  dotprod20/1 -> Mux/20
  "IW{1,1}(21,:)'"/1 -> dotprod21/1
  dotprod21/1 -> Mux/21
  "IW{1,1}(22,:)'"/1 -> dotprod22/1
  dotprod22/1 -> Mux/22
  "IW{1,1}(23,:)'"/1 -> dotprod23/1
  dotprod23/1 -> Mux/23
  "IW{1,1}(24,:)'"/1 -> dotprod24/1
  dotprod24/1 -> Mux/24
  "IW{1,1}(25,:)'"/1 -> dotprod25/1
  dotprod25/1 -> Mux/25
  "IW{1,1}(26,:)'"/1 -> dotprod26/1
  dotprod26/1 -> Mux/26
  "IW{1,1}(27,:)'"/1 -> dotprod27/1
  dotprod27/1 -> Mux/27
  "IW{1,1}(28,:)'"/1 -> dotprod28/1
  dotprod28/1 -> Mux/28
  "IW{1,1}(29,:)'"/1 -> dotprod29/1
  dotprod29/1 -> Mux/29
  "IW{1,1}(30,:)'"/1 -> dotprod30/1
  dotprod30/1 -> Mux/30
  Mux/1 -> "iz{1,1}"/1

== system mrefrobotarm_previous_y_previous_u_previous_ref_cex_3b/no_cex/Layer 2/Delays 1 ==
  "p{2}" : Inport  PortDimensions=30
      mask Display: e = 0.06;c1 = [120 230 180]/255;c2 = ([120 230 180]+0)/(256+128);c3 = ([120 230 180]+128)/(256+128);patch([0 1 1 0],[0 0 1 1],c1);patch([0 1 1 1-e 1-e 0+e],[0 0 1 1-e 0+e 0+e],c2);patch([0 0 1 1-e 0+e 0+e],[0 1 1 1-e 1-e 0+e],c3);plot([0 1 1 0 0],[0 0 1 1 0]);
  mux : Mux  Inputs=1
      mask Display: e = 0.06;c1 = [120 150 230]/255;c2 = ([120 150 230]+0)/383;c3 = ([120 150 230]+128)/383;patch([0 1 1 0],[0 0 1 1],c1);patch([0 1 1 1-e 1-e 0+e],[0 0 1 1-e 0+e 0+e],c2);patch([0 0 1 1-e 0+e 0+e],[0 1 1 1-e 1-e 0+e],c3);plot([0 1 1 0 0],[0 0 1 1 0]);disp('Mux')
  "pd{2,1}" : Outport
      mask Display: e = 0.06;c1 = [120 230 180]/255;c2 = ([120 230 180]+0)/(256+128);c3 = ([120 230 180]+128)/(256+128);patch([0 1 1 0],[0 0 1 1],c1);patch([0 1 1 1-e 1-e 0+e],[0 0 1 1-e 0+e 0+e],c2);patch([0 0 1 1-e 0+e 0+e],[0 1 1 1-e 1-e 0+e],c3);plot([0 1 1 0 0],[0 0 1 1 0]);
  wires:
  "p{2}"/1 -> mux/1
  mux/1 -> "pd{2,1}"/1
